simulink model "Test_thermal_transistor_Joul"  (R2022a)
settings: Solver=VariableStepAuto  StartTime=0.0  StopTime=200000  RelTol=1e-3
libraries: nesl_utility x8
settings Model: Creator=Ravi  LastModifiedBy=Ravi

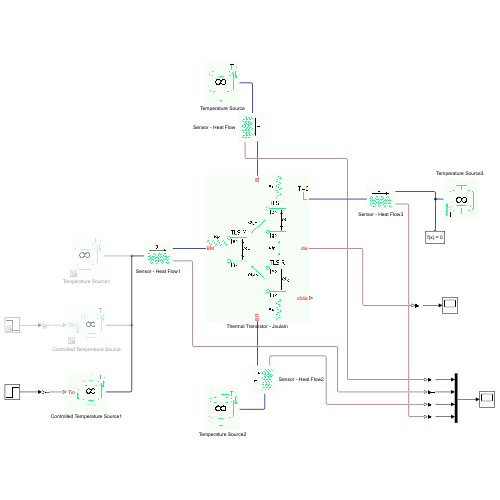
[thumbnail: Simulink's stored preview of the top-level diagram]
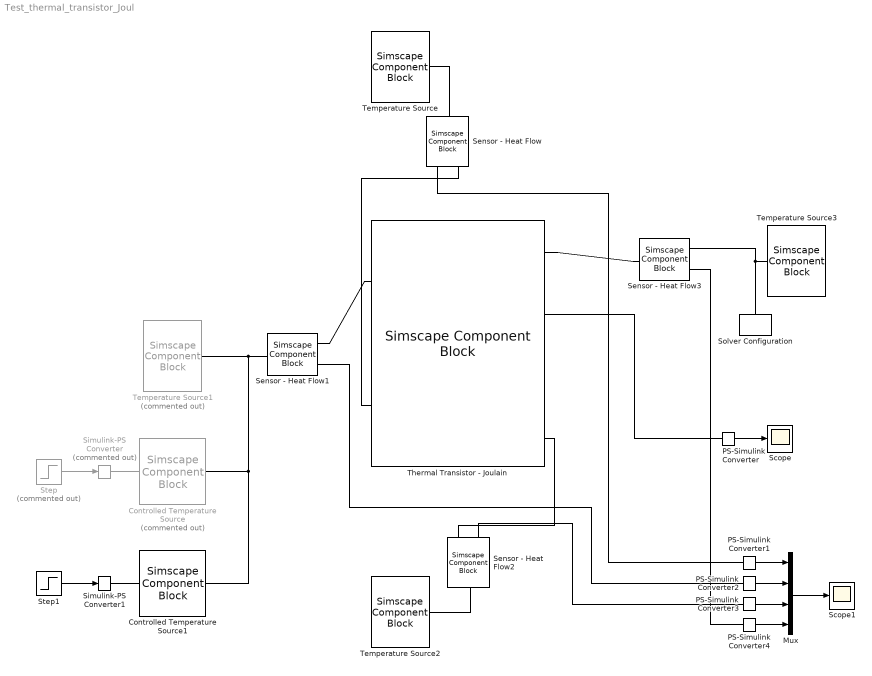
== system Test_thermal_transistor_Joul ==
  Controlled Temperature Source : SimscapeComponentBlock  Commented=on  SourceFile=source_controlled_temperature  ComponentPath=source_controlled_temperature  ComponentVariants="[\"source_controlled_temperature\"]"  ComponentVariantNames="[\"source_controlled_temperature\"]"  ClassName=source_controlled_temperature  SchemaVersion=1  J_specify=off  J_priority=None  J=0  J_nominal_specify=off  J_nominal_unit=1  J_nominal_value=1
      settings: CopyFcn=simscape.engine.sli.internal.componentblockcallback(gcbh,'COPY')  PreCopyFcn=simscape.engine.sli.internal.componentblockcallback(gcbh,'PRECOPY')  PreDeleteFcn=simscape.engine.sli.internal.componentblockcallback(gcbh,'PREDELETE')  InternalSimscapePortConfiguration="{\"Bottom\":[],\"Left\":[{\"id\":\"Tin\",\"label\":\"Tin\",\"type\":\"input\"}],\"Right\":[{\"id\":\"out\",\"label\":\"\",\"type\":\"quantum_thermal\"}],\"Top\":[]}"
      mask Type: Controlled temperature source
  Controlled Temperature Source1 : SimscapeComponentBlock  SourceFile=source_controlled_temperature  ComponentPath=source_controlled_temperature  ComponentVariants="[\"source_controlled_temperature\"]"  ComponentVariantNames="[\"source_controlled_temperature\"]"  ClassName=source_controlled_temperature  SchemaVersion=1  J_specify=off  J_priority=None  J=0  J_nominal_specify=off  J_nominal_unit=1  J_nominal_value=1
      settings: CopyFcn=simscape.engine.sli.internal.componentblockcallback(gcbh,'COPY')  PreCopyFcn=simscape.engine.sli.internal.componentblockcallback(gcbh,'PRECOPY')  PreDeleteFcn=simscape.engine.sli.internal.componentblockcallback(gcbh,'PREDELETE')  InternalSimscapePortConfiguration="{\"Bottom\":[],\"Left\":[{\"id\":\"Tin\",\"label\":\"Tin\",\"type\":\"input\"}],\"Right\":[{\"id\":\"out\",\"label\":\"\",\"type\":\"quantum_thermal\"}],\"Top\":[]}"
      mask Type: Controlled temperature source
  Mux : Mux
  PS-Simulink Converter{,1..4} (5 alike) : nesl_utility/PS-Simulink Converter  PhysicalDomain=network_engine_domain  SubClassName=ps_output  LeftPortType=input  RightPortType=output  PseudoPeriodic=off  Frequencies=[]  VectorFormat=inherit  Unit=inherit  AffineConversion=off
      settings: SourceProductBaseCode=SS,PW,VE
  Scope : Scope
  Scope1 : Scope
  Sensor - Heat Flow{,1..3} (4 alike) : SimscapeComponentBlock  SourceFile=sensor_heat_flow  ComponentPath=sensor_heat_flow  ComponentVariants="[\"sensor_heat_flow\"]"  ComponentVariantNames="[\"sensor_heat_flow\"]"  ClassName=sensor_heat_flow  SchemaVersion=1  J_specify=off  J_priority=None  J=0  J_nominal_specify=off  J_nominal_unit=1  J_nominal_value=1
      settings: CopyFcn=simscape.engine.sli.internal.componentblockcallback(gcbh,'COPY')  PreCopyFcn=simscape.engine.sli.internal.componentblockcallback(gcbh,'PRECOPY')  PreDeleteFcn=simscape.engine.sli.internal.componentblockcallback(gcbh,'PREDELETE')  InternalSimscapePortConfiguration="{\"Bottom\":[],\"Left\":[{\"id\":\"inp\",\"label\":\"\",\"type\":\"quantum_thermal\"}],\"Right\":[{\"id\":\"out\",\"label\":\"\",\"type\":\"quantum_thermal\"},{\"id\":\"sense\",\"label\":\"\",\"type\":\"output\"}],\"Top\":[]}"
      mask Type: Heat flow rate sensor
  Simulink-PS Converter : nesl_utility/Simulink-PS Converter  Commented=on  PhysicalDomain=network_engine_domain  SubClassName=ps_input  LeftPortType=input  RightPortType=output  PseudoPeriodic=off  Frequencies=[]  NoiseDistribution=none  NoiseParameters=[]  Unit=1  AffineConversion=off  FilteringAndDerivatives=provide  SimscapeFilterOrder=1  InputFilterTimeConstant=0.001  UdotUserProvided=0
      settings: SourceProductBaseCode=SS,PW,VE
  Simulink-PS Converter1 : nesl_utility/Simulink-PS Converter  PhysicalDomain=network_engine_domain  SubClassName=ps_input  LeftPortType=input  RightPortType=output  PseudoPeriodic=off  Frequencies=[]  NoiseDistribution=none  NoiseParameters=[]  Unit=1  AffineConversion=off  FilteringAndDerivatives=provide  SimscapeFilterOrder=1  InputFilterTimeConstant=0.001  UdotUserProvided=0
      settings: SourceProductBaseCode=SS,PW,VE
  Solver Configuration : nesl_utility/Solver Configuration  PhysicalDomain=network_engine_domain  SubClassName=solver  LeftPortType=input  RightPortType=generic  Tones=[]  Harmonics=[]  SimulateNoise=off  Profile=off  UseLocalSampling=off  EnableSwitchedLinearOptims=on  FrequencyDomain=off  UseCCode=off  RelTol=0.001  AbsTol=0.001  MinStep=1e-09  ToWorkspace=off  RevertToSquareIcSolve=off  NumHomotopyIterations=100  PhasorMode=off  PhasorModeNumHarmonics=1  IndexReductionMethod=DerivativeReplacement  DoDC=off  ResidualTolerance=1e-09  UseLocalSolver=off  LocalSolverChoice=NE_BACKWARD_EULER_ADVANCER  LocalSolverSampleTime=0.001  DoFixedCost=off  MaxNonlinIter=3  MaxModeIter=2  ComputeImpulses=off  ImpulseIterations=2  LinearAlgebra=auto  LinearAlgebraNumThread=0  EquationFormulation=NE_TIME_EF  DelaysMemoryBudget=1024  AutomaticFiltering=on  FilteringTimeConstant=0.001  PartitionStorageMethod=AS_NEEDED  PartitionMemoryBudget=1024  PartitionMethod=ROBUST
      settings: SourceProductBaseCode=SS,PW,VE
  Step : Step  Commented=on  Time=100000  Before=0.2  After=0.02  SampleTime=0
  Step1 : Step  Time=100000  Before=0.02  After=0.2  SampleTime=0
  Temperature Source : SimscapeComponentBlock  SourceFile=source_temperature  ComponentPath=source_temperature  ComponentVariants="[\"source_temperature\"]"  ComponentVariantNames="[\"source_temperature\"]"  ClassName=source_temperature  SchemaVersion=1  temp=0.2  J_specify=off  J_priority=None  J=0  J_nominal_specify=off  J_nominal_unit=1  J_nominal_value=1
      settings: CopyFcn=simscape.engine.sli.internal.componentblockcallback(gcbh,'COPY')  PreCopyFcn=simscape.engine.sli.internal.componentblockcallback(gcbh,'PRECOPY')  PreDeleteFcn=simscape.engine.sli.internal.componentblockcallback(gcbh,'PREDELETE')  InternalSimscapePortConfiguration="{\"Bottom\":[],\"Left\":[],\"Right\":[{\"id\":\"out\",\"label\":\"\",\"type\":\"quantum_thermal\"}],\"Top\":[]}"
      mask Type: Temperature source
  Temperature Source1 : SimscapeComponentBlock  Commented=on  SourceFile=source_temperature  ComponentPath=source_temperature  ComponentVariants="[\"source_temperature\"]"  ComponentVariantNames="[\"source_temperature\"]"  ClassName=source_temperature  SchemaVersion=1  temp=0.15  J_specify=off  J_priority=None  J=0  J_nominal_specify=off  J_nominal_unit=1  J_nominal_value=1
      settings: CopyFcn=simscape.engine.sli.internal.componentblockcallback(gcbh,'COPY')  PreCopyFcn=simscape.engine.sli.internal.componentblockcallback(gcbh,'PRECOPY')  PreDeleteFcn=simscape.engine.sli.internal.componentblockcallback(gcbh,'PREDELETE')  InternalSimscapePortConfiguration="{\"Bottom\":[],\"Left\":[],\"Right\":[{\"id\":\"out\",\"label\":\"\",\"type\":\"quantum_thermal\"}],\"Top\":[]}"
      mask Type: Temperature source
  Temperature Source2 : SimscapeComponentBlock  SourceFile=source_temperature  ComponentPath=source_temperature  ComponentVariants="[\"source_temperature\"]"  ComponentVariantNames="[\"source_temperature\"]"  ClassName=source_temperature  SchemaVersion=1  temp=0.02  J_specify=off  J_priority=None  J=0  J_nominal_specify=off  J_nominal_unit=1  J_nominal_value=1
      settings: CopyFcn=simscape.engine.sli.internal.componentblockcallback(gcbh,'COPY')  PreCopyFcn=simscape.engine.sli.internal.componentblockcallback(gcbh,'PRECOPY')  PreDeleteFcn=simscape.engine.sli.internal.componentblockcallback(gcbh,'PREDELETE')  InternalSimscapePortConfiguration="{\"Bottom\":[],\"Left\":[],\"Right\":[{\"id\":\"out\",\"label\":\"\",\"type\":\"quantum_thermal\"}],\"Top\":[]}"
      mask Type: Temperature source
  Temperature Source3 : SimscapeComponentBlock  SourceFile=source_temperature  ComponentPath=source_temperature  ComponentVariants="[\"source_temperature\"]"  ComponentVariantNames="[\"source_temperature\"]"  ClassName=source_temperature  SchemaVersion=1  temp=0  J_specify=off  J_priority=None  J=0  J_nominal_specify=off  J_nominal_unit=1  J_nominal_value=1
      settings: CopyFcn=simscape.engine.sli.internal.componentblockcallback(gcbh,'COPY')  PreCopyFcn=simscape.engine.sli.internal.componentblockcallback(gcbh,'PRECOPY')  PreDeleteFcn=simscape.engine.sli.internal.componentblockcallback(gcbh,'PREDELETE')  InternalSimscapePortConfiguration="{\"Bottom\":[],\"Left\":[],\"Right\":[{\"id\":\"out\",\"label\":\"\",\"type\":\"quantum_thermal\"}],\"Top\":[]}"
      mask Type: Temperature source
  Thermal Transistor - Joulain : SimscapeComponentBlock  SourceFile=thermal_transistor_Joul  ComponentPath=thermal_transistor_Joul  ComponentVariants="[\"thermal_transistor_Joul\"]"  ComponentVariantNames="[\"thermal_transistor_Joul\"]"  ClassName=thermal_transistor_Joul  SchemaVersion=1  kL=0.01  kM=0.01  kR=0.01  wL=0.0  wM=0.1  wR=0.0  wLM=1  wMR=1  wRL=0  p11_specify=off  p11_priority=High  p11=0.125  p11_nominal_specify=off  p11_nominal_unit=1  p11_nominal_value=1  p22_specify=off  p22_priority=High  p22=0.125  p22_nominal_specify=off  p22_nominal_unit=1  p22_nominal_value=1  p33_specify=off  p33_priority=High  p33=0.125  p33_nominal_specify=off  p33_nominal_unit=1  p33_nominal_value=1  p44_specify=off  p44_priority=High  p44=0.125  p44_nominal_specify=off  p44_nominal_unit=1  p44_nominal_value=1  p55_specify=off  p55_priority=High  p55=0.125  p55_nominal_specify=off  p55_nominal_unit=1  p55_nominal_value=1  p66_specify=off  p66_priority=High  p66=0.125  p66_nominal_specify=off  p66_nominal_unit=1  p66_nominal_value=1  p77_specify=off  p77_priority=High  p77=0.125  p77_nominal_specify=off  p77_nominal_unit=1  p77_nominal_value=1  p88_specify=off  p88_priority=High  p88=0.125  p88_nominal_specify=off  p88_nominal_unit=1  p88_nominal_value=1  TL_specify=off  TL_priority=Low  TL=0.2  TL_nominal_specify=off  TL_nominal_unit=1  TL_nominal_value=1  TM_specify=off  TM_priority=Low  TM=0.2  TM_nominal_specify=off  TM_nominal_unit=1  TM_nominal_value=1  TR_specify=off  TR_priority=Low  TR=0.2  TR_nominal_specify=off  TR_nominal_unit=1  TR_nominal_value=1  JL_specify=off  JL_priority=Low  JL=0  JL_nominal_specify=off  JL_nominal_unit=1  JL_nominal_value=1  JM_specify=off  JM_priority=Low  JM=0  JM_nominal_specify=off  JM_nominal_unit=1  JM_nominal_value=1  JR_specify=off  JR_priority=Low  JR=0  JR_nominal_specify=off  JR_nominal_unit=1  JR_nominal_value=1
      settings: CopyFcn=simscape.engine.sli.internal.componentblockcallback(gcbh,'COPY')  PreCopyFcn=simscape.engine.sli.internal.componentblockcallback(gcbh,'PRECOPY')  PreDeleteFcn=simscape.engine.sli.internal.componentblockcallback(gcbh,'PREDELETE')  InternalSimscapePortConfiguration="{\"Bottom\":[{\"id\":\"bR\",\"label\":\"BR\",\"type\":\"quantum_thermal\"}],\"Left\":[{\"id\":\"bM\",\"label\":\"BM\",\"type\":\"quantum_thermal\"}],\"Right\":[{\"id\":\"gnd\",\"label\":\"\",\"type\":\"quantum_thermal\"},{\"id\":\"diag\",\"label\":\"dia\",\"type\":\"output\"},{\"id\":\"ofdiag\",\"label\":\"ofdia\",\"type\":\"output\"}],\"Top\":[{\"id\":\"bL\",\"label\":\"BL\",\"type\":\"quantum_thermal\"}]}"
      mask Type: Thermal transistor
  wires:
  PS-Simulink Converter/1 -> Scope/1
  Mux/1 -> Scope1/1
  PS-Simulink Converter1/1 -> Mux/1
  PS-Simulink Converter2/1 -> Mux/2
  PS-Simulink Converter3/1 -> Mux/3
  PS-Simulink Converter4/1 -> Mux/4
  Step/1 -> Simulink-PS Converter/1
  Step1/1 -> Simulink-PS Converter1/1
  connections:
  Solver Configuration/RConn1 -- Sensor - Heat Flow3/RConn1 -- Temperature Source3/RConn1
  Sensor - Heat Flow2/RConn1 -- Thermal Transistor - Joulain/RConn4
  Temperature Source2/RConn1 -- Sensor - Heat Flow2/LConn1
  Sensor - Heat Flow1/RConn1 -- Thermal Transistor - Joulain/LConn1
  Sensor - Heat Flow/RConn1 -- Thermal Transistor - Joulain/LConn2
  Sensor - Heat Flow/LConn1 -- Temperature Source/RConn1
  PS-Simulink Converter/LConn1 -- Thermal Transistor - Joulain/RConn2
  Sensor - Heat Flow/RConn2 -- PS-Simulink Converter1/LConn1
  Sensor - Heat Flow1/RConn2 -- PS-Simulink Converter2/LConn1
  PS-Simulink Converter3/LConn1 -- Sensor - Heat Flow2/RConn2
  Thermal Transistor - Joulain/RConn1 -- Sensor - Heat Flow3/LConn1
  PS-Simulink Converter4/LConn1 -- Sensor - Heat Flow3/RConn2
  Controlled Temperature Source/LConn1 -- Simulink-PS Converter/RConn1
  Controlled Temperature Source1/RConn1 -- Controlled Temperature Source/RConn1 -- Sensor - Heat Flow1/LConn1 -- Temperature Source1/RConn1
  Controlled Temperature Source1/LConn1 -- Simulink-PS Converter1/RConn1
